simulink model "Obiekt_z_regulatorem"  (R2024b)
settings: Solver=VariableStepAuto  StartTime=0.0  StopTime=10.0  MaxStep=1  RelTol=1e-3
values from neighbouring files (symbols this model uses):
  c_p = 1000    [uklad_regulacji.m]
  C_vp = c_p*p_p*V_wp    (= 75000)    [uklad_regulacji.m]
  C_vw = c_p*p_p*V_we    (= 300000)    [uklad_regulacji.m]
  czas_skok = 1000    [uklad_regulacji.m]
  dPg = 1000    [uklad_regulacji.m]
  dSP = 2    [uklad_regulacji.m]
  dTzew = 0    [uklad_regulacji.m]
  f_pN = 0.01    [uklad_regulacji.m]
  K_1 = (0.6*P_gN)/(T_wewn-T_zewn)    (= 150)    [uklad_regulacji.m]
  K_d = (K_p*(T_wewn-T_pn))/(T_pn-T_zewn)    (= 100.571428571)    [uklad_regulacji.m]
  K_p = (P_gN-K_1*(T_wewn-T_zewn)-c_p*p_p*f_pN*(T_wewn-T_zewn))/(T_wewn-T_pn)    (= 704)    [uklad_regulacji.m]
  K_rp = 0.9*T/(K*T_0)    [uklad_regulacji.m]
  P_gN0 = P_gN*1    (= 10000)    [uklad_regulacji.m]
  p_p = 1.2    [uklad_regulacji.m]
  SP0 = T_pn    (= 15)    [uklad_regulacji.m]
  T_i = 3.33*T_0    (= 333)    [uklad_regulacji.m]
  T_p0 = (K_p*(T_wewn0)+K_d*T_zewn0)/(K_p+K_d)    (= 15)    [uklad_regulacji.m]
  T_wewn0 = T_zewn0 + (P_gN0)/(K_1+c_p*p_p*f_pN0+(K_p*K_d)/(K_p+K_d))    (= 20)    [uklad_regulacji.m]
  T_zewn0 = T_zewn+0    (= -20)    [uklad_regulacji.m]
settings Model: Creator=userbrigh  LastModifiedBy=userbrigh

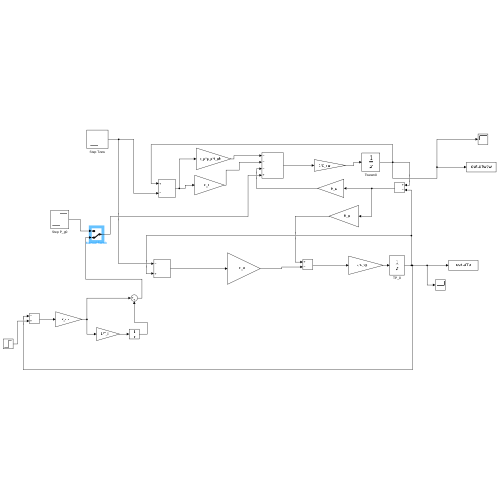
[thumbnail: Simulink's stored preview of the top-level diagram]
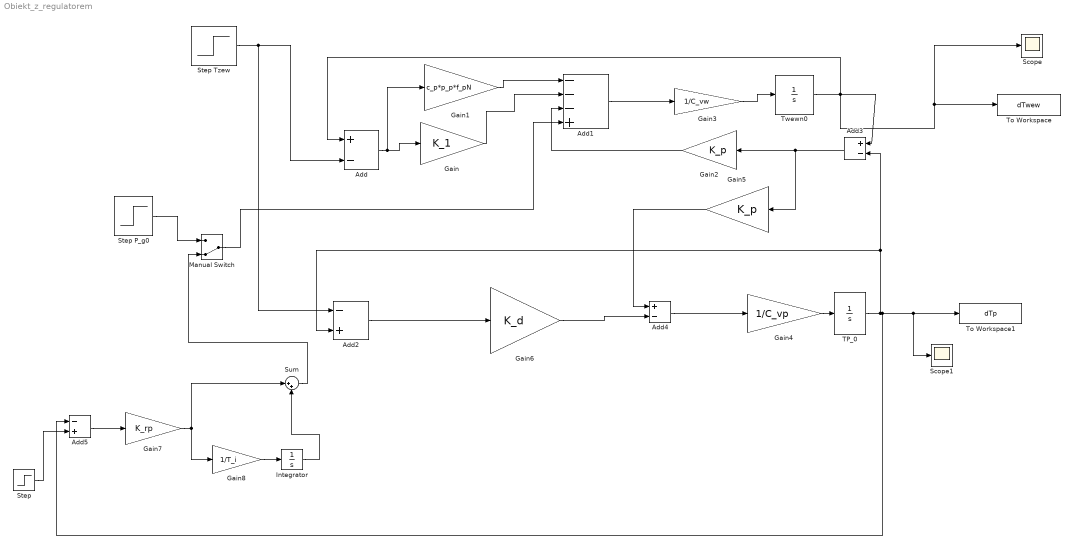
== system Obiekt_z_regulatorem ==
  Add : Sum  Inputs=+-
  Add1 : Sum  Inputs=---+
  Add2 : Sum  Inputs=-+
  Add3 : Sum  Inputs=+-
  Add4 : Sum  Inputs=+-
  Add5 : Sum  Inputs=-+
  Gain : Gain  Gain=K_1
  Gain1 : Gain  Gain=c_p*p_p*f_pN
  Gain2 : Gain  Gain=K_p
  Gain3 : Gain  Gain=1/C_vw
  Gain4 : Gain  Gain=1/C_vp
  Gain5 : Gain  Gain=K_p
  Gain6 : Gain  Gain=K_d
  Gain7 : Gain  Gain=K_rp
  Gain8 : Gain  Gain=1/T_i
  Integrator : Integrator  InitialCondition=P_gN0
  Manual Switch : ManualSwitch  CurrentSetting=0
  Scope : Scope
  Scope1 : Scope
  Step : Step  Time=czas_skok  Before=SP0  After=SP0+dSP  SampleTime=0
  Step P_g0 : Step  Time=czas_skok  Before=P_gN0  After=P_gN0+dPg  SampleTime=0
  Step Tzew : Step  Time=czas_skok  Before=T_zewn0  After=T_zewn0+dTzew  SampleTime=0
  Sum : Sum  Inputs=|++
  TP_0 : Integrator  InitialCondition=T_p0
  To Workspace : ToWorkspace  VariableName=dTwew  SampleTime=-1
  To Workspace1 : ToWorkspace  VariableName=dTp  SampleTime=-1
  Twewn0 : Integrator  InitialCondition=T_wewn0
  wires:
  Twewn0/1 -> Scope/1, To Workspace/1, Add/1, Add3/1
  Add3/1 -> Gain5/1, Gain2/1
  Step Tzew/1 -> Add2/1, Add/2
  Add/1 -> Gain1/1, Gain/1
  Gain/1 -> Add1/2
  Gain1/1 -> Add1/1
  Add1/1 -> Gain3/1
  Gain2/1 -> Add1/3
  Add2/1 -> Gain6/1
  Gain4/1 -> TP_0/1
  Gain3/1 -> Twewn0/1
  Gain5/1 -> Add4/1
  Gain6/1 -> Add4/2
  Add4/1 -> Gain4/1
  Step/1 -> Add5/2
  Integrator/1 -> Sum/2
  Add5/1 -> Gain7/1
  Gain7/1 -> Sum/1, Gain8/1
  Gain8/1 -> Integrator/1
  Step P_g0/1 -> Manual Switch/1
  Manual Switch/1 -> Add1/4
  Sum/1 -> Manual Switch/2
  TP_0/1 -> Add2/2, Add3/2, Scope1/1, To Workspace1/1, Add5/1
